simulink model "P6_CDCD_simulink"  (R2023b)
settings: Solver=ode23  StartTime=0.0  StopTime=0.010  RelTol=1e-3
values from neighbouring files (symbols this model uses):
  C = 10e-6    (= 1e-05)    [P6_CDCD.m]    (also in P6_CDCD_parameters.mat)
  d = 0.4    [P6_CDCD.m]    (also in P6_CDCD_parameters.mat)
  L = 2e-3    (= 0.002)    [P6_CDCD.m]    (also in P6_CDCD_parameters.mat)
  R = 10    [P6_CDCD.m]    (also in P6_CDCD_parameters.mat)

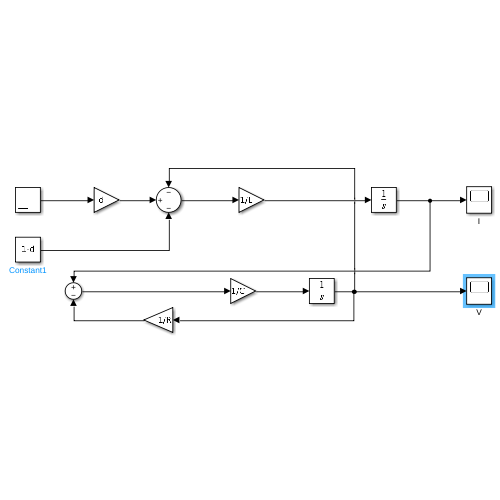
[thumbnail: Simulink's stored preview of the top-level diagram]
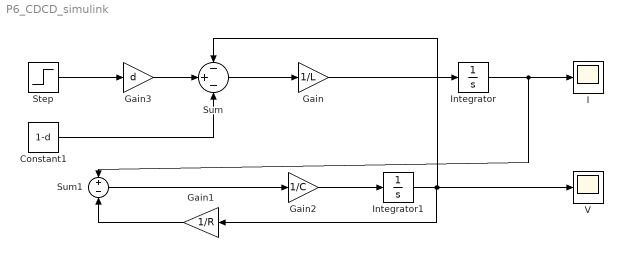
== system P6_CDCD_simulink ==
  Constant1 : Constant  Value=1-d
  Gain : Gain  Gain=1/L
  Gain1 : Gain  Gain=1/R
  Gain2 : Gain  Gain=1/C
  Gain3 : Gain  Gain=d
  I : Scope
  Integrator : Integrator
  Integrator1 : Integrator
  Step : Step  Time=0  After=32  SampleTime=0
  Sum : Sum  Inputs=-+-
  Sum1 : Sum  Inputs=+-
  V : Scope
  wires:
  Gain/1 -> Integrator/1
  Sum/1 -> Gain/1
  Gain2/1 -> Integrator1/1
  Integrator1/1 -> V/1, Sum/1, Gain1/1
  Step/1 -> Gain3/1
  Gain3/1 -> Sum/2
  Sum1/1 -> Gain2/1
  Gain1/1 -> Sum1/2
  Constant1/1 -> Sum/3
  Integrator/1 -> Sum1/1, I/1
